simulink model "SGA__suspension_skyhook_quarter"  (Simulink 7.2)
settings: Solver=ode45  StartTime=0.0  StopTime=10  RelTol=1e-3
libraries: simulink x2
settings Model: Creator=yichen  LastModifiedBy=yichen
settings OptimizationCC: BooleanDataType=off  InitFltsAndDblsToZero=on
settings DebuggingCC: SaveWithParameterizedLinksMsg=none  SignalResolutionControl=TryResolveAllWithWarning  SolverPrmCheckMsg=none  MultiTaskDSMMsg=warning  MultiTaskCondExecSysMsg=none  StrictBusMsg=None
settings HardwareCC: TargetUnknown=on
settings RTWCC: IncludeERTFirstTime=on
settings GRTTargetCC: TargetFcnLib=ansi_tfl_tmw.mat

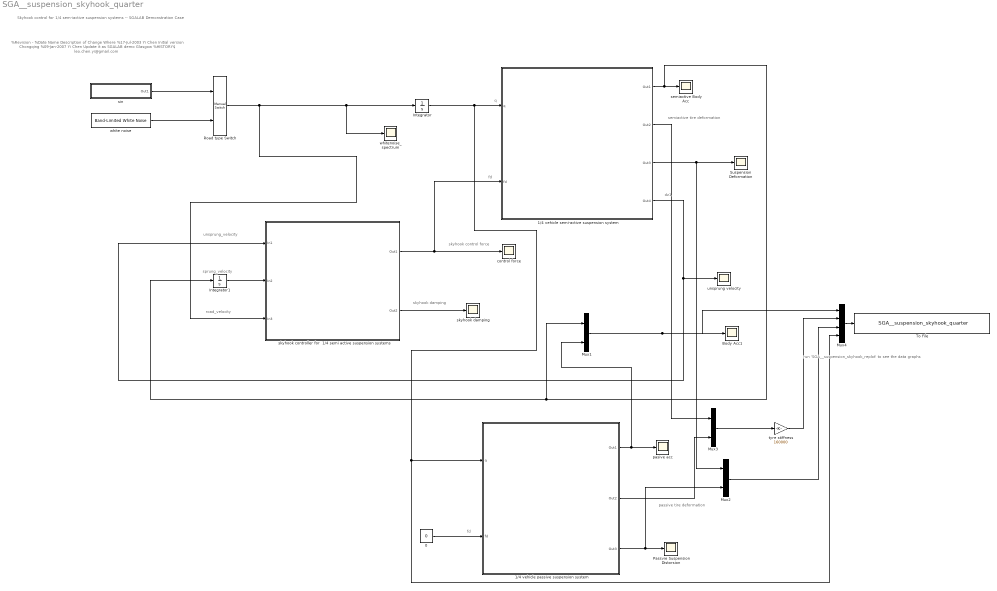
== system SGA__suspension_skyhook_quarter ==
  note: q
  note: fd
  note: unsprung_velocity
  note: sprung_velocity
  note: road_velocity
  note: skyhook control force
  note: skyhook damping
  note: dz1
  note: Skyhook control for 1/4 sem-iactive suspension systems
      | -- SGALAB Demonstration Case
  note: %Revision -
      | %Date                  Name        Description of Change                             Where
      | %17-Jul-2003     Yi Chen     Initial version                                              Chongqing
      | %09-Jan-2007    Yi Chen     Update it as SGALAB demo                     Glasgow
      | %HISTORY$  leo.chen.yi@gmail.com
  note: fd
  note: run 'SGA__suspension_skyhook_replot'
      | to see the data graphs
  note: passive tire deformation
  note: semiactive tire deformation
  " white noise" : simulink/Sources/Band-Limited White Noise  SystemSampleTime=-1  Cov=[256*10^-6]  Ts=0.01  seed=[23341]
  0 : Constant  Value=0  OutDataType=sfix(16)  OutScaling=2^0
  1/4 vehicle passive suspension system : Subsystem  mask{m1=36, m2=240, k1=160000, k2=16000, c0=1400, fr=300, g=9.8}
      mask prompts: m1 "Sprung mass-m1(kg)"; m2 "Unsprung mass-m2(kg)"; k1 "Stiffness of tyre-k1(N/m)"; k2 "Stiffness of suspension-k2(N/m)"; c0 "Coefficient of damper-c0(N/m/s)"; fr "Friction of suspension-fr(N)"; g "Acceleration of gravity-g(m/s^2)"
      mask help:
      | 1/4 passive vehicle suspension system
      | leo.chen.yi@gmail.com
      mask Display: image(imread('SGA__suspension_quarter_passive.jpg'));
  1/4 vehicle semi-active suspension system : Subsystem  mask{m1=36, m2=240, k1=160000, k2=16000, c0=1400, fr=300, g=9.8}
      mask prompts: m1 "Sprung mass-m1(kg)"; m2 "Unsprung mass-m2(kg"; k1 "Stiffness of tyre-k1(N/m)"; k2 "Stiffness of suspension-k2(N/m)"; c0 "Coefficient of damper-c0(N/m/s)"; fr "Friction of suspension-fr(N)"; g "Acceleration of gravity-g(m/s^2)"
      mask help:
      | 1/4 semi-active vehicle suspension system
      | leo.chen.yi@gmail.com
      mask Display: image(imread('SGA__suspension_quarter_passive.jpg'));
  Body Acc1 : Scope
      settings: YMin=-2.25  YMax=1.5  SaveName=ScopeData11
  Integrator : Integrator
  Integrator1 : Integrator
  Mux1 : Mux  Inputs=2
  Mux2 : Mux  Inputs=2
  Mux3 : Mux  Inputs=2
  Mux4 : Mux
  Passvie Suspension Distorsion : Scope
      settings: SaveName=ScopeData8
  Road type Switch : simulink/Signal Routing/Manual Switch  SystemSampleTime=-1  sw=1  action=0  varsize=off
  Suspension Deformation : Scope
      settings: SaveName=ScopeData2
  To File : ToFile  Filename=SGA__suspension_skyhook_quarter  MatrixName=SGA__suspension_skyhook_quarter
  control force : Scope
      settings: YMin=-2.5e+276  YMax=1.75e+277  SaveName=ScopeData3
  pasive acc : Scope
      settings: YMin=-2  YMax=2  SaveName=ScopeData10
  semiactive Body Acc : Scope
      settings: YMin=-2.25  YMax=2.5
  sin : Subsystem
      mask Display: disp('Sin Roadspectrum')
  skyhook controller for  1/4 semi active suspension systems : Subsystem
      mask Display: image(imread('SGA__suspension_skyhook_quarter.jpg'));
  skyhook damping : Scope
      settings: YMin=1000  YMax=3000  SaveName=ScopeData4
  tyre stiffness : Gain  Gain=160000  ParameterDataType=sfix(16)  ParameterScaling=2^0  OutDataType=sfix(16)  OutScaling=2^0  SaturateOnIntegerOverflow=on  OutDataTypeStr=Inherit: Same as input  ParamDataTypeStr=Inherit: Same as input
  unsprung velocity : Scope
      settings: YMin=-22.5  YMax=22.5  SaveName=ScopeData6
  whitenoise_spectrum : Scope
      settings: SaveName=ScopeData7
  wires:
  Road type Switch/1 -> whitenoise_spectrum/1, Integrator/1, skyhook controller for  1/4 semi active suspension systems/3(In3)
  1/4 vehicle semi-active suspension system/1(Out1) -> semiactive Body Acc/1, Integrator1/1, Mux1/1
  1/4 vehicle semi-active suspension system/3(Out3) -> Suspension Deformation/1, Mux2/1
  1/4 vehicle semi-active suspension system/2(Out2) -> Mux3/1
  skyhook controller for  1/4 semi active suspension systems/1(Out1) -> control force/1, 1/4 vehicle semi-active suspension system/2(fd)
  skyhook controller for  1/4 semi active suspension systems/2(Out2) -> skyhook damping/1
  1/4 vehicle semi-active suspension system/4(Out4) -> unsprung velocity/1, skyhook controller for  1/4 semi active suspension systems/1(In1)
  Integrator1/1 -> skyhook controller for  1/4 semi active suspension systems/2(In2)
  Integrator/1 -> 1/4 vehicle semi-active suspension system/1(q), 1/4 vehicle passive suspension system/1(q), Mux4/4
  1/4 vehicle passive suspension system/1(Out1) -> pasive acc/1, Mux1/2
  1/4 vehicle passive suspension system/3(Out3) -> Passvie Suspension Distorsion/1, Mux2/2
  1/4 vehicle passive suspension system/2(Out2) -> Mux3/2
  sin/1(Out1) -> Road type Switch/1
  " white noise"/1 -> Road type Switch/2
  0/1 -> 1/4 vehicle passive suspension system/2(fd)
  Mux4/1 -> To File/1
  Mux1/1 -> Body Acc1/1, Mux4/1
  Mux3/1 -> tyre stiffness/1
  tyre stiffness/1 -> Mux4/2
  Mux2/1 -> Mux4/3

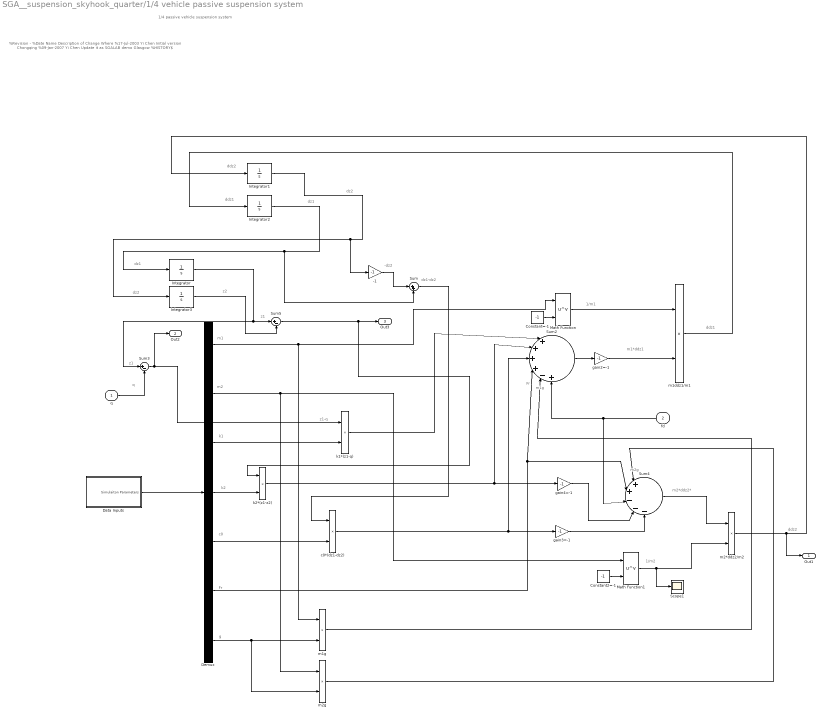
== system SGA__suspension_skyhook_quarter/1/4 vehicle passive suspension system ==
  note: m1
  note: k1
  note: m2
  note: k2
  note: c0
  note: z1
  note: dz1
  note: Fr
  note: g
  note: dz2
  note: -dz2
  note: dz1-dz2
  note: dz1
  note: dz2
  note: ddz2
  note: q
  note: z1
  note: z1-q
  note: Fr
  note: m1g
  note: m1*ddz1
  note: 1/m1
  note: ddz1
  note: m2g
  note: m2*ddz2*
  note: 1/m2
  note: ddz2
  note: z2
  note: ddz1
  note: 1/4 passive vehicle suspension system
  note: %Revision -
      | %Date                  Name        Description of Change                             Where
      | %17-Jul-2003     Yi Chen     Initial version                                              Chongqing
      | %09-Jan-2007    Yi Chen     Update it as SGALAB demo                    Glasgow
      | %HISTORY$
  q : Inport  OutDataType=sfix(16)  OutScaling=2^0
  fd : Inport  Orientation=left  Port=2  OutDataType=sfix(16)  OutScaling=2^0
  -1 : Gain  Gain=-1  ParameterDataType=sfix(16)  ParameterScaling=2^0  OutDataType=sfix(16)  OutScaling=2^0  SaturateOnIntegerOverflow=on  OutDataTypeStr=Inherit: Same as input  ParamDataTypeStr=Inherit: Same as input
  Constant2=-1 : Constant  Value=-1  OutDataType=sfix(16)  OutScaling=2^0
  Constant=-1 : Constant  Value=-1  OutDataType=sfix(16)  OutScaling=2^0
  Data Inputs : Subsystem
  Demux : Demux  Outputs=7  BusSelectionMode=on
  Integrator{,1..3} (4 alike) : Integrator
  Math Function : Math  Operator=pow  OutDataType=sfix(16)  OutScaling=2^0  SaturateOnIntegerOverflow=on
  Math Function1 : Math  Operator=pow  OutDataType=sfix(16)  OutScaling=2^0  SaturateOnIntegerOverflow=on
  Scope1 : Scope
      settings: SaveName=ScopeData5
  Sum : Sum  Inputs=|++  OutDataType=sfix(16)  OutScaling=2^0  SaturateOnIntegerOverflow=on  InputSameDT=on  OutDataTypeStr=Inherit: Same as first input
  Sum2 : Sum  Inputs=|++++-+  OutDataType=sfix(16)  OutScaling=2^0  SaturateOnIntegerOverflow=on  InputSameDT=on  OutDataTypeStr=Inherit: Same as first input
  Sum3 : Sum  Inputs=|+-  OutDataType=sfix(16)  OutScaling=2^0  SaturateOnIntegerOverflow=on  InputSameDT=on  OutDataTypeStr=Inherit: Same as first input
  Sum4 : Sum  Inputs=|++---  OutDataType=sfix(16)  OutScaling=2^0  SaturateOnIntegerOverflow=on  InputSameDT=on  OutDataTypeStr=Inherit: Same as first input
  Sum5 : Sum  Inputs=|+-  OutDataType=sfix(16)  OutScaling=2^0  SaturateOnIntegerOverflow=on  InputSameDT=on  OutDataTypeStr=Inherit: Same as first input
  c0*(dz1-dz2) : Product  OutDataType=sfix(16)  OutScaling=2^0  SaturateOnIntegerOverflow=on  RndMeth=Zero  InputSameDT=on  OutDataTypeStr=Inherit: Same as first input
  gain2=-1 : Gain  Gain=-1  ParameterDataType=sfix(16)  ParameterScaling=2^0  OutDataType=sfix(16)  OutScaling=2^0  SaturateOnIntegerOverflow=on  OutDataTypeStr=Inherit: Same as input  ParamDataTypeStr=Inherit: Same as input
  gain3=-1 : Gain  Gain=-1  ParameterDataType=sfix(16)  ParameterScaling=2^0  OutDataType=sfix(16)  OutScaling=2^0  SaturateOnIntegerOverflow=on  OutDataTypeStr=Inherit: Same as input  ParamDataTypeStr=Inherit: Same as input
  gain4=-1 : Gain  Gain=-1  ParameterDataType=sfix(16)  ParameterScaling=2^0  OutDataType=sfix(16)  OutScaling=2^0  SaturateOnIntegerOverflow=on  OutDataTypeStr=Inherit: Same as input  ParamDataTypeStr=Inherit: Same as input
  k1*(z1-q) : Product  OutDataType=sfix(16)  OutScaling=2^0  SaturateOnIntegerOverflow=on  RndMeth=Zero  InputSameDT=on  OutDataTypeStr=Inherit: Same as first input
  k2*(z1-z2) : Product  OutDataType=sfix(16)  OutScaling=2^0  SaturateOnIntegerOverflow=on  RndMeth=Zero  InputSameDT=on  OutDataTypeStr=Inherit: Same as first input
  m1ddz1/m1 : Product  OutDataType=sfix(16)  OutScaling=2^0  SaturateOnIntegerOverflow=on  RndMeth=Zero  InputSameDT=on  OutDataTypeStr=Inherit: Same as first input
  m1g : Product  OutDataType=sfix(16)  OutScaling=2^0  SaturateOnIntegerOverflow=on  RndMeth=Zero  InputSameDT=on  OutDataTypeStr=Inherit: Same as first input
  m2*ddz2/m2 : Product  OutDataType=sfix(16)  OutScaling=2^0  SaturateOnIntegerOverflow=on  RndMeth=Zero  InputSameDT=on  OutDataTypeStr=Inherit: Same as first input
  m2g : Product  OutDataType=sfix(16)  OutScaling=2^0  SaturateOnIntegerOverflow=on  RndMeth=Zero  InputSameDT=on  OutDataTypeStr=Inherit: Same as first input
  Out1 : Outport  OutDataType=sfix(16)  OutScaling=2^0
  Out2 : Outport  Port=2  OutDataType=sfix(16)  OutScaling=2^0
  Out3 : Outport  Port=3  OutDataType=sfix(16)  OutScaling=2^0
  wires:
  Data Inputs/1("Simulaiton Parameters ") -> Demux/1
  Demux/1 -> m1g/1, Math Function/1
  Integrator2/1 -> Sum/2, Integrator/1
  Integrator/1 -> Sum5/1, Sum3/1
  Demux/5 -> c0*(dz1-dz2)/2
  -1/1 -> Sum/1
  Sum/1 -> c0*(dz1-dz2)/1
  Integrator1/1 -> -1/1, Integrator3/1
  Demux/4 -> k2*(z1-z2)/2
  Demux/3 -> k1*(z1-q)/2
  Sum3/1 -> k1*(z1-q)/1, Out2/1
  Sum2/1 -> gain2=-1/1
  gain2=-1/1 -> m1ddz1/m1/2
  k1*(z1-q)/1 -> Sum2/1
  k2*(z1-z2)/1 -> Sum2/2, gain4=-1/1
  c0*(dz1-dz2)/1 -> Sum2/3, gain3=-1/1
  fd/1 -> Sum2/6, Sum4/3
  Constant=-1/1 -> Math Function/2
  Math Function/1 -> m1ddz1/m1/1
  m1ddz1/m1/1 -> Integrator2/1
  Demux/6 -> Sum2/4, Sum4/2
  gain3=-1/1 -> Sum4/5
  gain4=-1/1 -> Sum4/4
  Sum4/1 -> m2*ddz2/m2/1
  Demux/7 -> m1g/2, m2g/2
  Demux/2 -> m2g/1, Math Function1/1
  m1g/1 -> Sum2/5
  m2g/1 -> Sum4/1
  Constant2=-1/1 -> Math Function1/2
  Math Function1/1 -> m2*ddz2/m2/2, Scope1/1
  m2*ddz2/m2/1 -> Integrator1/1, Out1/1
  Integrator3/1 -> Sum5/2
  Sum5/1 -> k2*(z1-z2)/1, Out3/1
  q/1 -> Sum3/2

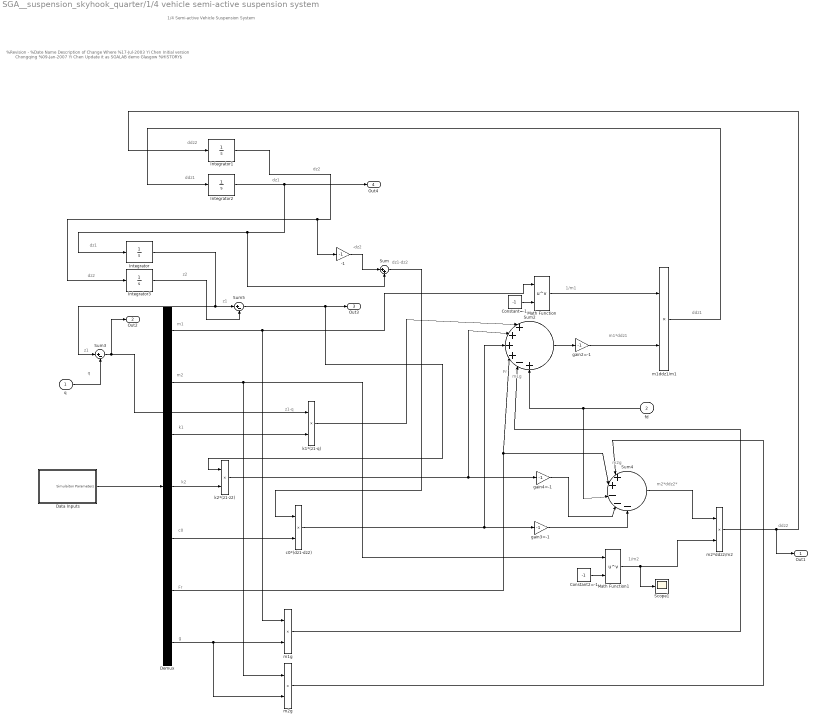
== system SGA__suspension_skyhook_quarter/1/4 vehicle semi-active suspension system ==
  note: m1
  note: k1
  note: m2
  note: k2
  note: c0
  note: z1
  note: dz1
  note: Fr
  note: g
  note: dz2
  note: -dz2
  note: dz1-dz2
  note: dz1
  note: dz2
  note: ddz2
  note: q
  note: z1
  note: z1-q
  note: Fr
  note: m1g
  note: m1*ddz1
  note: 1/m1
  note: ddz1
  note: m2g
  note: m2*ddz2*
  note: 1/m2
  note: ddz2
  note: z2
  note: ddz1
  note: 1/4 Semi-active Vehicle Suspension System
  note: %Revision -
      | %Date                  Name        Description of Change                             Where
      | %17-Jul-2003     Yi Chen     Initial version                                              Chongqing
      | %09-Jan-2007    Yi Chen     Update it as SGALAB demo                    Glasgow
      | %HISTORY$
  q : Inport  OutDataType=sfix(16)  OutScaling=2^0
  fd : Inport  Orientation=left  Port=2  OutDataType=sfix(16)  OutScaling=2^0
  -1 : Gain  Gain=-1  ParameterDataType=sfix(16)  ParameterScaling=2^0  OutDataType=sfix(16)  OutScaling=2^0  SaturateOnIntegerOverflow=on  OutDataTypeStr=Inherit: Same as input  ParamDataTypeStr=Inherit: Same as input
  Constant2=-1 : Constant  Value=-1  OutDataType=sfix(16)  OutScaling=2^0
  Constant=-1 : Constant  Value=-1  OutDataType=sfix(16)  OutScaling=2^0
  Data Inputs : Subsystem
  Demux : Demux  Outputs=7  BusSelectionMode=on
  Integrator{,1..3} (4 alike) : Integrator
  Math Function : Math  Operator=pow  OutDataType=sfix(16)  OutScaling=2^0  SaturateOnIntegerOverflow=on
  Math Function1 : Math  Operator=pow  OutDataType=sfix(16)  OutScaling=2^0  SaturateOnIntegerOverflow=on
  Scope1 : Scope
      settings: SaveName=ScopeData5
  Sum : Sum  Inputs=|++  OutDataType=sfix(16)  OutScaling=2^0  SaturateOnIntegerOverflow=on  InputSameDT=on  OutDataTypeStr=Inherit: Same as first input
  Sum2 : Sum  Inputs=|++++-+  OutDataType=sfix(16)  OutScaling=2^0  SaturateOnIntegerOverflow=on  InputSameDT=on  OutDataTypeStr=Inherit: Same as first input
  Sum3 : Sum  Inputs=|+-  OutDataType=sfix(16)  OutScaling=2^0  SaturateOnIntegerOverflow=on  InputSameDT=on  OutDataTypeStr=Inherit: Same as first input
  Sum4 : Sum  Inputs=|++---  OutDataType=sfix(16)  OutScaling=2^0  SaturateOnIntegerOverflow=on  InputSameDT=on  OutDataTypeStr=Inherit: Same as first input
  Sum5 : Sum  Inputs=|+-  OutDataType=sfix(16)  OutScaling=2^0  SaturateOnIntegerOverflow=on  InputSameDT=on  OutDataTypeStr=Inherit: Same as first input
  c0*(dz1-dz2) : Product  OutDataType=sfix(16)  OutScaling=2^0  SaturateOnIntegerOverflow=on  RndMeth=Zero  InputSameDT=on  OutDataTypeStr=Inherit: Same as first input
  gain2=-1 : Gain  Gain=-1  ParameterDataType=sfix(16)  ParameterScaling=2^0  OutDataType=sfix(16)  OutScaling=2^0  SaturateOnIntegerOverflow=on  OutDataTypeStr=Inherit: Same as input  ParamDataTypeStr=Inherit: Same as input
  gain3=-1 : Gain  Gain=-1  ParameterDataType=sfix(16)  ParameterScaling=2^0  OutDataType=sfix(16)  OutScaling=2^0  SaturateOnIntegerOverflow=on  OutDataTypeStr=Inherit: Same as input  ParamDataTypeStr=Inherit: Same as input
  gain4=-1 : Gain  Gain=-1  ParameterDataType=sfix(16)  ParameterScaling=2^0  OutDataType=sfix(16)  OutScaling=2^0  SaturateOnIntegerOverflow=on  OutDataTypeStr=Inherit: Same as input  ParamDataTypeStr=Inherit: Same as input
  k1*(z1-q) : Product  OutDataType=sfix(16)  OutScaling=2^0  SaturateOnIntegerOverflow=on  RndMeth=Zero  InputSameDT=on  OutDataTypeStr=Inherit: Same as first input
  k2*(z1-z2) : Product  OutDataType=sfix(16)  OutScaling=2^0  SaturateOnIntegerOverflow=on  RndMeth=Zero  InputSameDT=on  OutDataTypeStr=Inherit: Same as first input
  m1ddz1/m1 : Product  OutDataType=sfix(16)  OutScaling=2^0  SaturateOnIntegerOverflow=on  RndMeth=Zero  InputSameDT=on  OutDataTypeStr=Inherit: Same as first input
  m1g : Product  OutDataType=sfix(16)  OutScaling=2^0  SaturateOnIntegerOverflow=on  RndMeth=Zero  InputSameDT=on  OutDataTypeStr=Inherit: Same as first input
  m2*ddz2/m2 : Product  OutDataType=sfix(16)  OutScaling=2^0  SaturateOnIntegerOverflow=on  RndMeth=Zero  InputSameDT=on  OutDataTypeStr=Inherit: Same as first input
  m2g : Product  OutDataType=sfix(16)  OutScaling=2^0  SaturateOnIntegerOverflow=on  RndMeth=Zero  InputSameDT=on  OutDataTypeStr=Inherit: Same as first input
  Out1 : Outport  OutDataType=sfix(16)  OutScaling=2^0
  Out2 : Outport  Port=2  OutDataType=sfix(16)  OutScaling=2^0
  Out3 : Outport  Port=3  OutDataType=sfix(16)  OutScaling=2^0
  Out4 : Outport  Port=4  OutDataType=sfix(16)  OutScaling=2^0
  wires:
  Data Inputs/1("Simulaiton Parameters ") -> Demux/1
  Demux/1 -> m1g/1, Math Function/1
  Integrator2/1 -> Sum/2, Integrator/1, Out4/1
  Integrator/1 -> Sum5/1, Sum3/1
  Demux/5 -> c0*(dz1-dz2)/2
  -1/1 -> Sum/1
  Sum/1 -> c0*(dz1-dz2)/1
  Integrator1/1 -> -1/1, Integrator3/1
  Demux/4 -> k2*(z1-z2)/2
  Demux/3 -> k1*(z1-q)/2
  Sum3/1 -> k1*(z1-q)/1, Out2/1
  Sum2/1 -> gain2=-1/1
  gain2=-1/1 -> m1ddz1/m1/2
  k1*(z1-q)/1 -> Sum2/1
  k2*(z1-z2)/1 -> Sum2/2, gain4=-1/1
  c0*(dz1-dz2)/1 -> Sum2/3, gain3=-1/1
  fd/1 -> Sum2/6, Sum4/3
  Constant=-1/1 -> Math Function/2
  Math Function/1 -> m1ddz1/m1/1
  m1ddz1/m1/1 -> Integrator2/1
  Demux/6 -> Sum2/4, Sum4/2
  gain3=-1/1 -> Sum4/5
  gain4=-1/1 -> Sum4/4
  Sum4/1 -> m2*ddz2/m2/1
  Demux/7 -> m1g/2, m2g/2
  Demux/2 -> m2g/1, Math Function1/1
  m1g/1 -> Sum2/5
  m2g/1 -> Sum4/1
  Constant2=-1/1 -> Math Function1/2
  Math Function1/1 -> m2*ddz2/m2/2, Scope1/1
  m2*ddz2/m2/1 -> Integrator1/1, Out1/1
  Integrator3/1 -> Sum5/2
  Sum5/1 -> k2*(z1-z2)/1, Out3/1
  q/1 -> Sum3/2

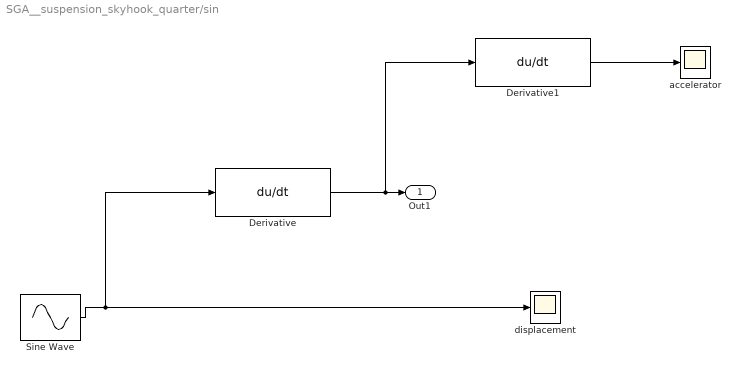
== system SGA__suspension_skyhook_quarter/sin ==
  Derivative : Derivative
  Derivative1 : Derivative
  Sine Wave : Sin  Amplitude=0.015  Frequency=2  SampleTime=0
  accelerator : Scope
      settings: SaveName=ScopeData2
  displacement : Scope
  Out1 : Outport  OutDataType=sfix(16)  OutScaling=2^0
  wires:
  Sine Wave/1 -> displacement/1, Derivative/1
  Derivative/1 -> Derivative1/1, Out1/1
  Derivative1/1 -> accelerator/1

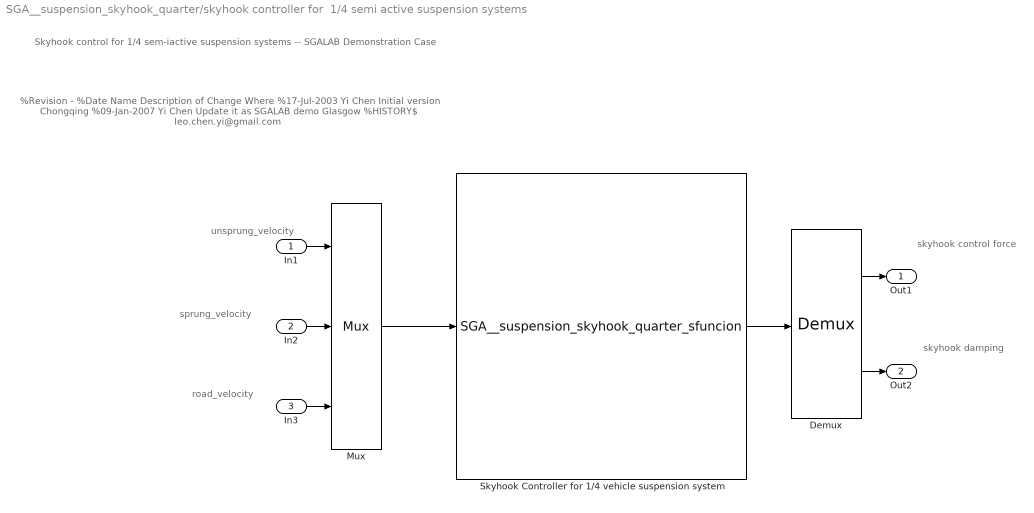
== system SGA__suspension_skyhook_quarter/skyhook controller for  1/4 semi active suspension systems ==
  note: unsprung_velocity
  note: sprung_velocity
  note: road_velocity
  note: skyhook control force
  note: skyhook damping
  note: Skyhook control for 1/4 sem-iactive suspension systems
      | -- SGALAB Demonstration Case
  note: %Revision -
      | %Date                  Name        Description of Change                             Where
      | %17-Jul-2003     Yi Chen     Initial version                                              Chongqing
      | %09-Jan-2007    Yi Chen     Update it as SGALAB demo                     Glasgow
      | %HISTORY$  leo.chen.yi@gmail.com
  In1 : Inport  OutDataType=sfix(16)  OutScaling=2^0
  In2 : Inport  Port=2  OutDataType=sfix(16)  OutScaling=2^0
  In3 : Inport  Port=3  OutDataType=sfix(16)  OutScaling=2^0
  " Skyhook Controller for 1/4 vehicle suspension system" : S-Function  Description=Practical skyhook controller  FunctionName=SGA__suspension_skyhook_quarter_sfuncion  Parameters=Cfirm,Csoft,Csh  EnableBusSupport=off  mask{Cfirm=3000, Csoft=1000, Csh=1800}
      mask prompts: Cfirm "Max Damping Of Skyhook"; Csoft "Min Damping Of skyhook"; Csh "Expecting Damping Of Skyhook"
      mask help:
      | Pratical Skyhook controller for semi active suspension systems
      |
      |     if ( Cfirm/Csh ) < Sprung_Velocity/(Unsprung_Velocity-Sprung_Velocity)
      |
      |           u_control             = Cfirm*(Unsprung_Velocity-Sprung_Velocity);
      |           c_semi_skyhook = Cfirm;
      |
      |     elseif (Csoft/Csh) < Sprung_Velocity/(Unsprung_Velocity-Sprung_Velocity)&(Cfirm/Csh)>Sprung_Velocity/(Unsprung_Velocity-Sprung_Velocity)
      |
      |           u_control            =  Csh*Sprung_Velocity;
      |           c_semi_skyhook = Csh*Sprung_Velocity/(Unsprung_Velocity-Sprung_Velocity);
      |
      |     else
      |
      |         u_control             = Csoft*(Unsprung_Velocity-Sprung_Velocity);
      |         c_semi_skyhook = Csoft;
      |
      |     end
      mask Help:
      | Skyhook control for 1/4 sem-iactive suspension systems
      | -- SGALAB Demonstration Case
      | %Revision -
      | %Date                  Name        Description of Change                             Where
      | %17-Jul-2003     Yi Chen     Initial version                                              Chongqing
      | %09-Jan-2007    Yi Chen     Update it as SGALAB demo                     Glasgow
      | %HISTORY$  leo.chen.yi@gmail.com
      mask Display: image(imread('SGA__suspension_skyhook_quater.jpg'));
  Demux : Demux  Outputs=2
  Mux : Mux  Inputs=3
      settings: DisplayOption=signals
  Out1 : Outport  OutDataType=sfix(16)  OutScaling=2^0
  Out2 : Outport  Port=2  OutDataType=sfix(16)  OutScaling=2^0
  wires:
  Mux/1 -> " Skyhook Controller for 1/4 vehicle suspension system"/1
  " Skyhook Controller for 1/4 vehicle suspension system"/1 -> Demux/1
  In1/1 -> Mux/1
  Demux/1 -> Out1/1
  In2/1 -> Mux/2
  Demux/2 -> Out2/1
  In3/1 -> Mux/3

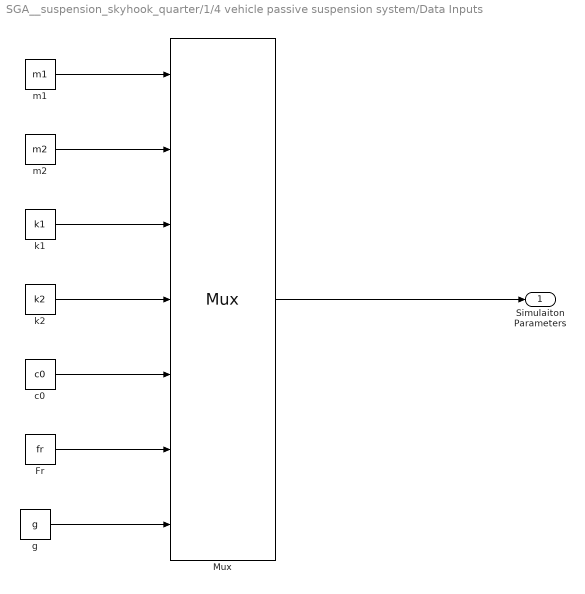
== system SGA__suspension_skyhook_quarter/1/4 vehicle passive suspension system/Data Inputs ==
  Fr : Constant  Value=fr  OutDataType=sfix(16)  OutScaling=2^0
  Mux : Mux  Inputs=7
  c0 : Constant  Value=c0  OutDataType=sfix(16)  OutScaling=2^0
  g : Constant  Value=g  OutDataType=sfix(16)  OutScaling=2^0
  k1 : Constant  Value=k1  OutDataType=sfix(16)  OutScaling=2^0
  k2 : Constant  Value=k2  OutDataType=sfix(16)  OutScaling=2^0
  m1 : Constant  Value=m1  OutDataType=sfix(16)  OutScaling=2^0
  m2 : Constant  Value=m2  OutDataType=sfix(16)  OutScaling=2^0
  "Simulaiton Parameters " : Outport  OutDataType=sfix(16)  OutScaling=2^0
  wires:
  m1/1 -> Mux/1
  m2/1 -> Mux/2
  k1/1 -> Mux/3
  k2/1 -> Mux/4
  c0/1 -> Mux/5
  Fr/1 -> Mux/6
  g/1 -> Mux/7
  Mux/1 -> "Simulaiton Parameters "/1

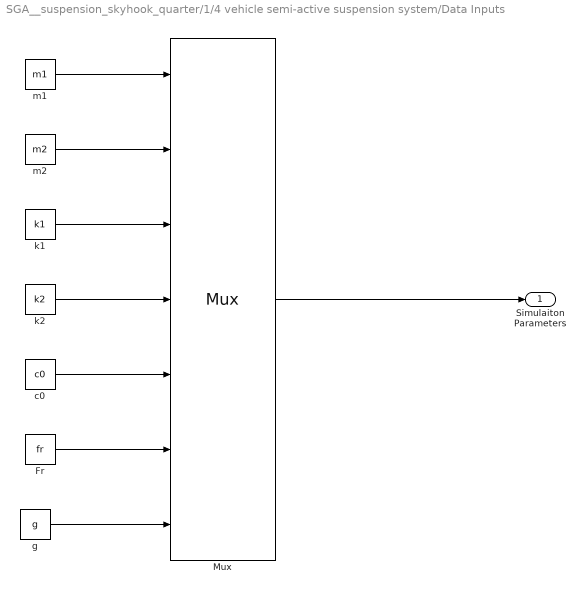
== system SGA__suspension_skyhook_quarter/1/4 vehicle semi-active suspension system/Data Inputs ==
  Fr : Constant  Value=fr  OutDataType=sfix(16)  OutScaling=2^0
  Mux : Mux  Inputs=7
  c0 : Constant  Value=c0  OutDataType=sfix(16)  OutScaling=2^0
  g : Constant  Value=g  OutDataType=sfix(16)  OutScaling=2^0
  k1 : Constant  Value=k1  OutDataType=sfix(16)  OutScaling=2^0
  k2 : Constant  Value=k2  OutDataType=sfix(16)  OutScaling=2^0
  m1 : Constant  Value=m1  OutDataType=sfix(16)  OutScaling=2^0
  m2 : Constant  Value=m2  OutDataType=sfix(16)  OutScaling=2^0
  "Simulaiton Parameters " : Outport  OutDataType=sfix(16)  OutScaling=2^0
  wires:
  m1/1 -> Mux/1
  m2/1 -> Mux/2
  k1/1 -> Mux/3
  k2/1 -> Mux/4
  c0/1 -> Mux/5
  Fr/1 -> Mux/6
  g/1 -> Mux/7
  Mux/1 -> "Simulaiton Parameters "/1
